simulink model "Bai_2"  (R2023a)
settings: Solver=VariableStepAuto  StartTime=0.0  StopTime=10.0  RelTol=1e-3  EnableMultiTasking=on
libraries: simulink x3, dspfdesign x2, simulink_extras x2, dspsrcs4 x2
settings Model: Creator=Admin  LastModifiedBy=Admin
settings SolverCC: AlgebraicLoopSolver=TrustRegion
settings DataIOCC: ReturnWorkspaceOutputs=off
settings OptimizationCC: LifeSpan=inf
settings DebuggingCC: UnconnectedInputMsg=warning  UnconnectedOutputMsg=warning  UnconnectedLineMsg=warning  SFUnexpectedBacktrackingDiag=warning  SFNoUnconditionalDefaultTransitionDiag=warning  ArithmeticOperatorsInVariantConditions=warning
settings ModelReferenceCC: EnableRefExpFcnMdlSchedulingChecks=on
settings SFSimCC: SimUseLocalCustomCode=off  CustomCodeUndefinedFunction=UseInterfaceOnly
settings RTWCC: RTWUseLocalCustomCode=off
settings CodeAppCC: StateflowObjectComments=on
settings GRTTargetCC: TargetLangStandard=C89/C90 (ANSI)
settings ConfigComp: CovMetricSettings=dw  CovSaveCumulativeToWorkspaceVar=on  CovSaveSingleToWorkspaceVar=on  CovExternalEMLEnable=off

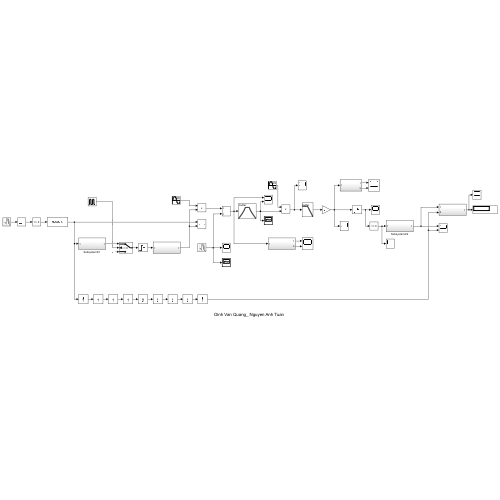
[thumbnail: Simulink's stored preview of the top-level diagram]
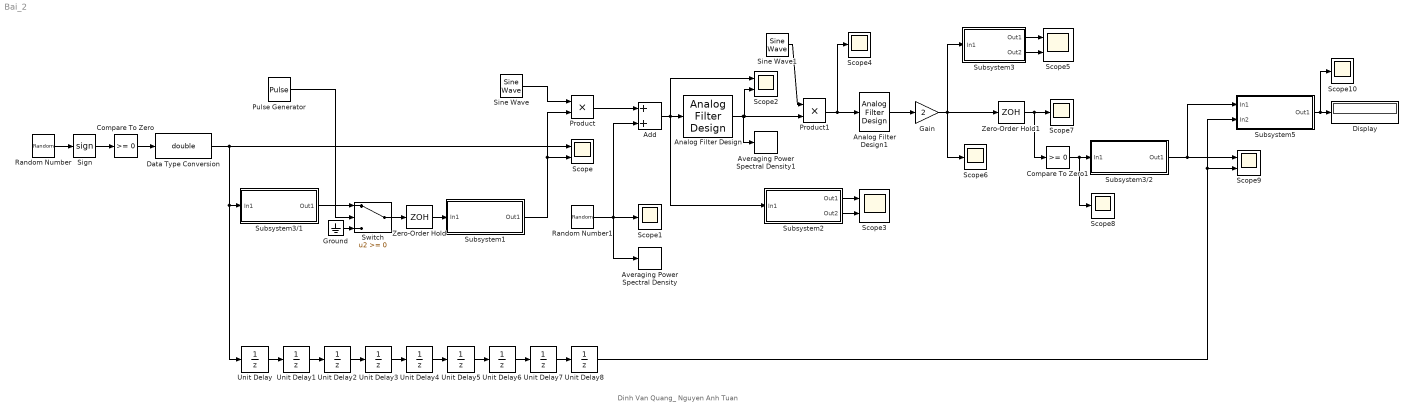
== system Bai_2 ==
  note: Dinh Van Quang_ Nguyen Anh Tuan
  Add : Sum
  Analog Filter Design : dspfdesign/Analog Filter Design  method=Butterworth  filttype=Bandpass  N=8  Wlo=30  Whi=80  Rp=2  Rs=40
  Analog Filter Design1 : dspfdesign/Analog Filter Design  method=Butterworth  filttype=Lowpass  N=8  Wlo=30  Whi=80  Rp=2  Rs=40
  Averaging Power Spectral Density : simulink_extras/Additional Sinks/Averaging Power Spectral Density  npts=128  fftpts=512  HowOften=64  sampleT=0.1
  Averaging Power Spectral Density1 : simulink_extras/Additional Sinks/Averaging Power Spectral Density  npts=128  fftpts=512  HowOften=64  sampleT=0.1
  Compare To Zero : simulink/Logic and Bit Operations/Compare To Zero  relop=>=  OutDataTypeStr=boolean
  Compare To Zero1 : simulink/Logic and Bit Operations/Compare To Zero  relop=>=  OutDataTypeStr=boolean
  Data Type Conversion : DataTypeConversion  OutDataTypeStr=double  SaturateOnIntegerOverflow=off  RndMeth=Floor
  Display : Display
  Gain : Gain  Gain=2
  Ground : Ground
  Product : Product
  Product1 : Product
  Pulse Generator : DiscretePulseGenerator  PulseType=Time based  Period=10  PulseWidth=5
  Random Number : RandomNumber  SampleTime=0.1
  Random Number1 : RandomNumber  SampleTime=0.1
  Scope{,2..3,5,9} (5 alike) : Scope  NumInputPorts=2
  Scope{1,4,6..8,10} (6 alike) : Scope
  Sign : Signum
  Sine Wave : dspsrcs4/Sine Wave  Amplitude=1  Frequency=15*pi  Phase=0  SampleMode=Discrete  OutComplex=Real  CompMethod=Trigonometric fcn  TableSize=Speed  SampleTime=1/1000  SamplesPerFrame=1  ResetState=Restart at time zero  OutputFrames=off  dataType=double  wordLen=16  udDataType=sfix(16)  fracBitsMode=Best precision  numFracBits=15  OutDataTypeStr=double  LastOutDataTypeStr=double
  Sine Wave1 : dspsrcs4/Sine Wave  Amplitude=1  Frequency=15*pi  Phase=0  SampleMode=Discrete  OutComplex=Real  CompMethod=Trigonometric fcn  TableSize=Speed  SampleTime=1/1000  SamplesPerFrame=1  ResetState=Restart at time zero  OutputFrames=off  dataType=double  wordLen=16  udDataType=sfix(16)  fracBitsMode=Best precision  numFracBits=15  OutDataTypeStr=double  LastOutDataTypeStr=double
  Subsystem1 : Subsystem
  Subsystem2 : Subsystem
  Subsystem3 : Subsystem
  Subsystem3/1 : Subsystem
  Subsystem3/2 : Subsystem
  Subsystem5 : Subsystem
  Switch : Switch  SaturateOnIntegerOverflow=off  InputSameDT=off
  Unit Delay{,1..8} (9 alike) : UnitDelay  SampleTime=-1  HasFrameUpgradeWarning=on
  Zero-Order Hold : ZeroOrderHold  SampleTime=-1
  Zero-Order Hold1 : ZeroOrderHold  SampleTime=-1
  wires:
  Random Number/1 -> Sign/1
  Sign/1 -> Compare To Zero/1
  Compare To Zero/1 -> Data Type Conversion/1
  Unit Delay/1 -> Unit Delay1/1
  Unit Delay1/1 -> Unit Delay2/1
  Unit Delay2/1 -> Unit Delay3/1
  Unit Delay3/1 -> Unit Delay4/1
  Unit Delay4/1 -> Unit Delay5/1
  Unit Delay5/1 -> Unit Delay6/1
  Unit Delay6/1 -> Unit Delay7/1
  Unit Delay7/1 -> Unit Delay8/1
  Subsystem3/1/1(Out1) -> Switch/1
  Switch/1 -> Zero-Order Hold/1
  Pulse Generator/1 -> Switch/2
  Zero-Order Hold/1 -> Subsystem1/1(In1)
  Data Type Conversion/1 -> Scope/1, Subsystem3/1/1(In1), Unit Delay/1
  Subsystem1/1(Out1) -> Scope/2, Product/2
  Sine Wave/1 -> Product/1
  Random Number1/1 -> Averaging Power Spectral Density/1, Add/2, Scope1/1
  Product/1 -> Add/1
  Add/1 -> Subsystem2/1(In1), Scope2/1, Analog Filter Design/1
  Sine Wave1/1 -> Product1/1
  Analog Filter Design/1 -> Averaging Power Spectral Density1/1, Scope2/2, Product1/2
  Subsystem2/1(Out1) -> Scope3/1
  Subsystem2/2(Out2) -> Scope3/2
  Product1/1 -> Scope4/1, Analog Filter Design1/1
  Gain/1 -> Scope6/1, Subsystem3/1(In1), Zero-Order Hold1/1
  Subsystem3/1(Out1) -> Scope5/1
  Subsystem3/2(Out2) -> Scope5/2
  Zero-Order Hold1/1 -> Compare To Zero1/1, Scope7/1
  Compare To Zero1/1 -> Subsystem3/2/1(In1), Scope8/1
  Subsystem3/2/1(Out1) -> Subsystem5/1(In1), Scope9/1
  Unit Delay8/1 -> Scope9/2, Subsystem5/2(In2)
  Subsystem5/1(Out1) -> Scope10/1, Display/1
  Ground/1 -> Switch/3
  Analog Filter Design1/1 -> Gain/1

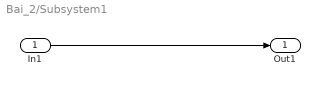
== system Bai_2/Subsystem1 ==
  In1 : Inport
  Out1 : Outport
  wires:
  In1/1 -> Out1/1

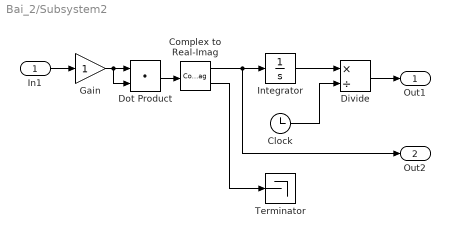
== system Bai_2/Subsystem2 ==
  In1 : Inport
  Clock : Clock
  Complex to Real-Imag : ComplexToRealImag
  Divide : Product  Inputs=*/
  Dot Product : DotProduct  OutDataTypeStr=Inherit: Inherit via internal rule
  Gain : Gain
  Integrator : Integrator
  Terminator : Terminator
  Out1 : Outport
  Out2 : Outport  Port=2
  wires:
  Gain/1 -> Dot Product/2, Dot Product/1
  In1/1 -> Gain/1
  Dot Product/1 -> Complex to Real-Imag/1
  Complex to Real-Imag/2 -> Terminator/1
  Complex to Real-Imag/1 -> Out2/1, Integrator/1
  Integrator/1 -> Divide/1
  Divide/1 -> Out1/1
  Clock/1 -> Divide/2

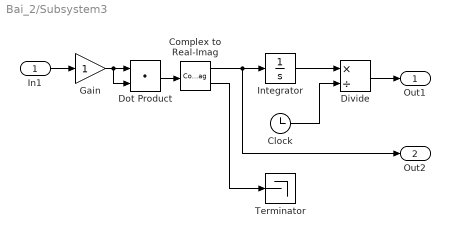
== system Bai_2/Subsystem3 ==
  In1 : Inport
  Clock : Clock
  Complex to Real-Imag : ComplexToRealImag
  Divide : Product  Inputs=*/
  Dot Product : DotProduct  OutDataTypeStr=Inherit: Inherit via internal rule
  Gain : Gain
  Integrator : Integrator
  Terminator : Terminator
  Out1 : Outport
  Out2 : Outport  Port=2
  wires:
  Gain/1 -> Dot Product/2, Dot Product/1
  In1/1 -> Gain/1
  Dot Product/1 -> Complex to Real-Imag/1
  Complex to Real-Imag/2 -> Terminator/1
  Complex to Real-Imag/1 -> Out2/1, Integrator/1
  Integrator/1 -> Divide/1
  Divide/1 -> Out1/1
  Clock/1 -> Divide/2

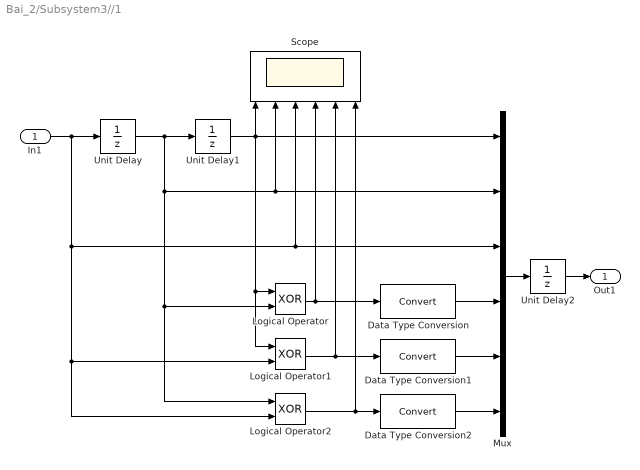
== system Bai_2/Subsystem3//1 ==
  In1 : Inport
  Data Type Conversion : DataTypeConversion  SaturateOnIntegerOverflow=off  RndMeth=Floor
  Data Type Conversion1 : DataTypeConversion  SaturateOnIntegerOverflow=off  RndMeth=Floor
  Data Type Conversion2 : DataTypeConversion  SaturateOnIntegerOverflow=off  RndMeth=Floor
  Logical Operator : Logic  Operator=XOR  AllPortsSameDT=off  OutDataTypeStr=boolean
  Logical Operator1 : Logic  Operator=XOR  AllPortsSameDT=off  OutDataTypeStr=boolean
  Logical Operator2 : Logic  Operator=XOR  AllPortsSameDT=off  OutDataTypeStr=boolean
  Mux : Mux  Inputs=6
  Scope : Scope  NumInputPorts=6
  Unit Delay : UnitDelay  SampleTime=-1  HasFrameUpgradeWarning=on
  Unit Delay1 : UnitDelay  SampleTime=-1  HasFrameUpgradeWarning=on
  Unit Delay2 : UnitDelay  SampleTime=-1  HasFrameUpgradeWarning=on
  Out1 : Outport
  wires:
  In1/1 -> Scope/3, Mux/3, Logical Operator1/2, Logical Operator2/2, Unit Delay/1
  Unit Delay/1 -> Scope/2, Mux/2, Logical Operator/2, Logical Operator2/1, Unit Delay1/1
  Unit Delay1/1 -> Scope/1, Mux/1, Logical Operator1/1, Logical Operator/1
  Logical Operator/1 -> Scope/4, Data Type Conversion/1
  Logical Operator1/1 -> Scope/5, Data Type Conversion1/1
  Logical Operator2/1 -> Scope/6, Data Type Conversion2/1
  Data Type Conversion2/1 -> Mux/6
  Data Type Conversion1/1 -> Mux/5
  Mux/1 -> Unit Delay2/1
  Unit Delay2/1 -> Out1/1
  Data Type Conversion/1 -> Mux/4

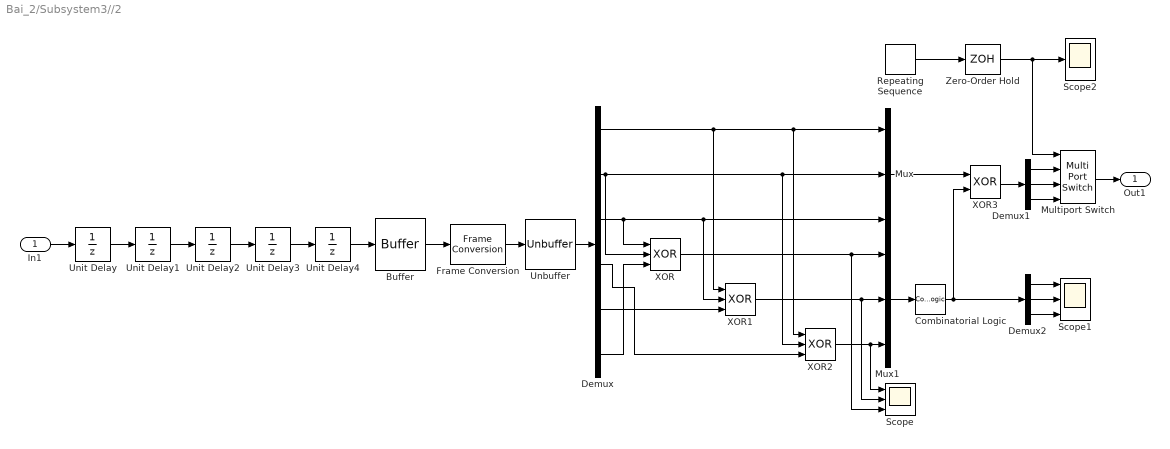
== system Bai_2/Subsystem3//2 ==
  In1 : Inport
  Buffer : Buffer  OutputFrames=off
  Combinatorial Logic : CombinatorialLogic
  Demux : Demux  Outputs=6
  Demux1 : Demux  Outputs=3
  Demux2 : Demux  Outputs=3
  Frame Conversion : FrameConversion  OutFrame=Sample-based
  Multiport Switch : MultiPortSwitch  SaturateOnIntegerOverflow=off  InputSameDT=off
  Mux : Mux  Inputs=3
  Mux1 : Mux  Inputs=3
  Repeating Sequence : simulink/Sources/Repeating Sequence  rep_seq_t=[0 2]  rep_seq_y=[0 2]
  Scope : Scope  NumInputPorts=3
  Scope1 : Scope  NumInputPorts=3
  Scope2 : Scope
  Unbuffer : Unbuffer
  Unit Delay{,1..4} (5 alike) : UnitDelay  SampleTime=-1  HasFrameUpgradeWarning=on
  XOR : Logic  Operator=XOR  Inputs=3  AllPortsSameDT=off  OutDataTypeStr=boolean
  XOR1 : Logic  Operator=XOR  Inputs=3  AllPortsSameDT=off  OutDataTypeStr=boolean
  XOR2 : Logic  Operator=XOR  Inputs=3  AllPortsSameDT=off  OutDataTypeStr=boolean
  XOR3 : Logic  Operator=XOR  AllPortsSameDT=off  OutDataTypeStr=boolean
  Zero-Order Hold : ZeroOrderHold  SampleTime=-1
  Out1 : Outport
  wires:
  In1/1 -> Unit Delay/1
  Unit Delay/1 -> Unit Delay1/1
  Unit Delay1/1 -> Unit Delay2/1
  Unit Delay2/1 -> Unit Delay3/1
  Unit Delay3/1 -> Unit Delay4/1
  Unit Delay4/1 -> Buffer/1
  Buffer/1 -> Frame Conversion/1
  Demux/2 -> XOR/2, XOR2/2, Mux/2
  Demux/1 -> XOR1/1, XOR2/1, Mux/1
  Demux/3 -> XOR/1, XOR1/2, Mux/3
  Demux/6 -> XOR/3
  Demux/5 -> XOR1/3
  Demux/4 -> XOR2/3
  XOR/1 -> Scope/3, Mux1/1
  XOR1/1 -> Scope/2, Mux1/2
  XOR2/1 -> Scope/1, Mux1/3
  Mux1/1 -> Combinatorial Logic/1
  Combinatorial Logic/1 -> Demux2/1, XOR3/2
  Mux/1 -> XOR3/1
  Repeating Sequence/1 -> Zero-Order Hold/1
  XOR3/1 -> Demux1/1
  Demux1/3 -> Multiport Switch/4
  Demux1/2 -> Multiport Switch/3
  Demux1/1 -> Multiport Switch/2
  Zero-Order Hold/1 -> Scope2/1, Multiport Switch/1
  Multiport Switch/1 -> Out1/1
  Demux2/2 -> Scope1/2
  Demux2/1 -> Scope1/1
  Demux2/3 -> Scope1/3
  Frame Conversion/1 -> Unbuffer/1
  Unbuffer/1 -> Demux/1

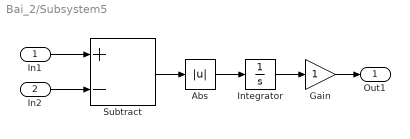
== system Bai_2/Subsystem5 ==
  In1 : Inport
  In2 : Inport  Port=2
  Abs : Abs  SaturateOnIntegerOverflow=off
  Gain : Gain
  Integrator : Integrator
  Subtract : Sum  Inputs=+-
  Out1 : Outport
  wires:
  In1/1 -> Subtract/1
  In2/1 -> Subtract/2
  Subtract/1 -> Abs/1
  Abs/1 -> Integrator/1
  Integrator/1 -> Gain/1
  Gain/1 -> Out1/1
